simulink model "lab_1"  (R2024b)
settings: Solver=FixedStepAuto  StartTime=0.0  StopTime=inf  FixedStep=0.001  RelTol=1e-3  EnableMultiTasking=on
libraries: stm32f4xxblockslib x16, simulink x15, stm32g4xxblockslib x6
settings Model: STM32="{\"AnalogInput\":[{\"ID\":\"lab_1:1\"},{\"ID\":\"lab_1:151\"},{\"ID\":\"lab_1:191\"}],\"DigitalPortRead\":[{\"ID\":\"lab_1:126\"},{\"ID\":\"lab_1:163\"},{\"ID\":\"lab_1:197\"},{\"ID\":\"lab_1:248\"},{\"ID\":\"lab_1:260\"},{\"ID\":\"lab_1:272\"},{\"ID\":\"lab_1:237\"},{\"ID\":\"lab_1:238\"},{\"ID\":\"lab_1:303\"},{\"ID\":\"lab_1:314\"},{\"ID\":\"lab_1:325\"},{\"ID\":\"lab_1:293\"},{\"ID\":\"lab_1:294\"}],\"EncoderBlockForG4\":[{\"ID\":\"lab_1:234\"},{\"ID\":\"lab_1:235\"},{\"ID\":\"lab_1:236\"},{\"ID\":\"lab_1:290\"},{\"ID\":\"lab_1:291\"},{\"ID\":\"lab_1:292\"}]}"  Creator=A1nz_01  LastModifiedBy=user
settings OptimizationCC: EnhancedBackFolding=on  PassReuseOutputArgsAs=Individual arguments  ZeroExternalMemoryAtStartup=off  ZeroInternalMemoryAtStartup=off  MaxStackSize=512  OptimizeBlockOrder=speed  DifferentSizesBufferReuse=on  OptimizationCustomize=off  EfficientTunableParamExpr=on
settings DebuggingCC: ParameterTunabilityLossMsg=error
settings HardwareCC: ProdBitPerPointer=32  ProdBitPerSizeT=32  ProdBitPerPtrDiffT=32  ProdLargestAtomicInteger=Long  ProdLargestAtomicFloat=Double  ProdWordSize=32  ProdLongLongMode=on  ProdHWDeviceType=ARM Compatible->ARM Cortex-M
settings SFSimCC: MATLABDynamicMemAlloc=off
settings RTWCC: Description=Embedded Coder  SystemTargetFile=ert.tlc  HardwareBoard=STM32G4xx Based  TemplateMakefile=ert_default_tmf  Toolchain=GNU Tools for ARM Embedded Processors
settings CodeAppCC: ForceParamTrailComments=on  IgnoreCustomStorageClasses=off  OperatorAnnotations=on  SimulinkDataObjDesc=on  SFDataObjDesc=on  InsertBlockDesc=on
settings ERTTargetCC: TargetLangStandard=C99 (ISO)  CodeReplacementLibrary=ARM Cortex-M  ExtModeTransport=3  ExtModeStaticAlloc=on  ExtModeStaticAllocSize=2048  ExtModeMexFile=ext_xcp  ExtModeIntrfLevel=Level2 - Open  InlinedParameterPlacement=Hierarchical  DynamicArrayContainerType=coder::array

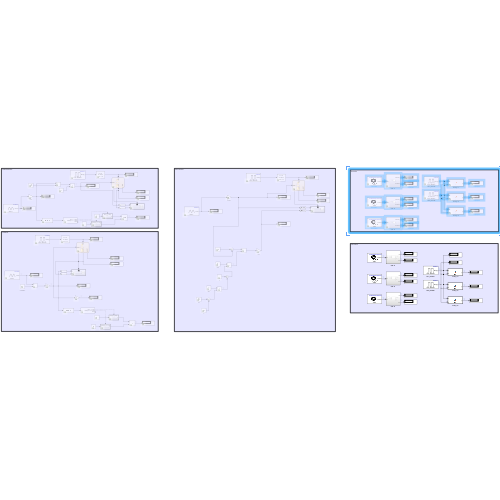
[thumbnail: Simulink's stored preview of the top-level diagram]
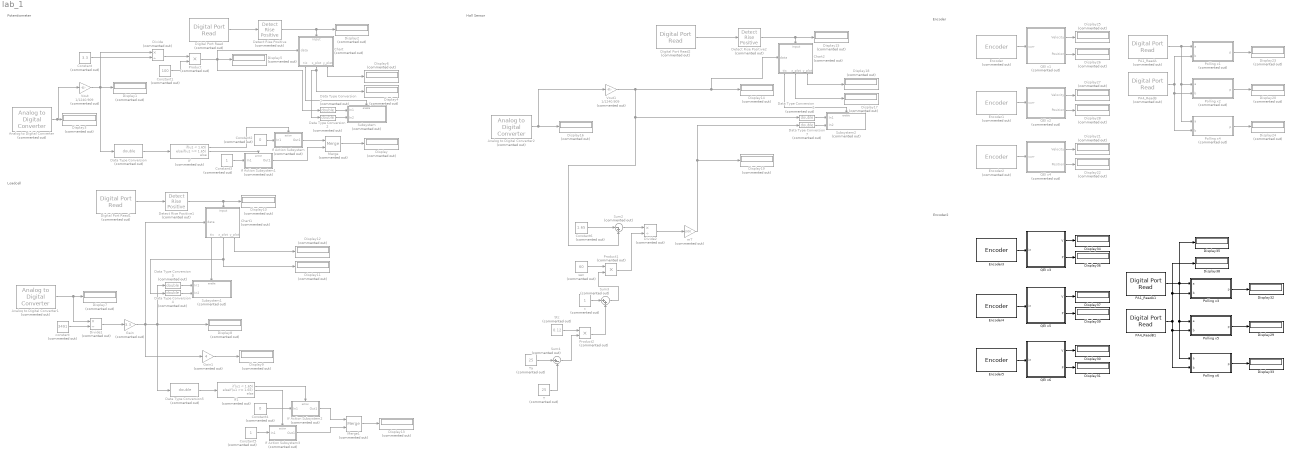
== system lab_1 ==
  note: Encoder2
  note: Encoder
  note: Hall Sensor
  note: Loadcell
  note: Potentiometer
  Analog to Digital Converter : stm32f4xxblockslib/Analog to Digital Converter  Commented=on  ADCModule=ADC1  ConversionGroup=Regular  TriggerMode=Trigger and read  NumberOfConversions=1  EnableBufferConv=off  BufferLength=1  OutputStatus=off  SampleTime=-1  EnableSimPort=off  hoistedMaskSrc=ECSoC/ECSimCodegen/Analog to Digital Converter
  Analog to Digital Converter1 : stm32f4xxblockslib/Analog to Digital Converter  Commented=on  ADCModule=ADC1  ConversionGroup=Regular  TriggerMode=Trigger and read  NumberOfConversions=1  EnableBufferConv=off  BufferLength=1  OutputStatus=off  SampleTime=-1  EnableSimPort=off  hoistedMaskSrc=ECSoC/ECSimCodegen/Analog to Digital Converter
  Analog to Digital Converter2 : stm32f4xxblockslib/Analog to Digital Converter  Commented=on  ADCModule=ADC1  ConversionGroup=Regular  TriggerMode=Trigger and read  NumberOfConversions=1  EnableBufferConv=off  BufferLength=1  OutputStatus=off  SampleTime=-1  EnableSimPort=off  hoistedMaskSrc=ECSoC/ECSimCodegen/Analog to Digital Converter
  Chart : Stateflow chart  Commented=on  TreatAsAtomicUnit=on
      settings: PortSchema="{\"entries\":[{\"content\":{\"sides\":[{\"content\":{\"connectorIds\":[\"In1\"]},\"type\":\"ConnectorPlacement.EquallySpacedRectSide\",\"uuid\":\"15421bba-938f-45a9-ad39-0fb1dc31f746\"},{\"content\":{\"side\":\"RIGHT\"},\"type\":\"ConnectorPlacement.EquallySpacedRectSide\",\"uuid\":\"6df644a9-cb47-4d86-919b-b55e97b0d3b9\"},{\"content\":{\"connectorIds\":[\"In2\"],\"side\":\"TOP\"},\"type\":\"ConnectorPlacement.EquallySpacedRectSide\",\"uuid\":\"9fcc37fd-4916-48d6-817c-74b5556d6fa8\"},{\"content\":{\"connectorIds\":[\"Out1\",\"Out2\",\"Out3\"],\"side\":\"BOTTOM\"},\"type\":\"ConnectorPlacement.EquallySpacedRectSide\",\"uuid\":\"cb540dc6-d65e-4d03-87d2-789e1aed4831\"}]},\"type\":\"ConnectorPlacement.EquallySpacedConnector\",\"uuid\":\"c07b23df-6d95-4e9d-8fab-891c31dfc579\"}],\"packageUris\":[\"http://schema.mathworks.com/mf0/Connector/R2020b\"],\"version\":\"1.0\"}"
  Chart1 : Stateflow chart  Commented=on  TreatAsAtomicUnit=on
      settings: PortSchema="{\"entries\":[{\"content\":{\"sides\":[{\"content\":{\"connectorIds\":[\"In1\"]},\"type\":\"ConnectorPlacement.EquallySpacedRectSide\",\"uuid\":\"15421bba-938f-45a9-ad39-0fb1dc31f746\"},{\"content\":{\"side\":\"RIGHT\"},\"type\":\"ConnectorPlacement.EquallySpacedRectSide\",\"uuid\":\"6df644a9-cb47-4d86-919b-b55e97b0d3b9\"},{\"content\":{\"connectorIds\":[\"In2\"],\"side\":\"TOP\"},\"type\":\"ConnectorPlacement.EquallySpacedRectSide\",\"uuid\":\"9fcc37fd-4916-48d6-817c-74b5556d6fa8\"},{\"content\":{\"connectorIds\":[\"Out1\",\"Out2\",\"Out3\"],\"side\":\"BOTTOM\"},\"type\":\"ConnectorPlacement.EquallySpacedRectSide\",\"uuid\":\"cb540dc6-d65e-4d03-87d2-789e1aed4831\"}]},\"type\":\"ConnectorPlacement.EquallySpacedConnector\",\"uuid\":\"c07b23df-6d95-4e9d-8fab-891c31dfc579\"}],\"packageUris\":[\"http://schema.mathworks.com/mf0/Connector/R2020b\"],\"version\":\"1.0\"}"
  Chart2 : Stateflow chart  Commented=on  TreatAsAtomicUnit=on
      settings: PortSchema="{\"entries\":[{\"content\":{\"sides\":[{\"content\":{\"connectorIds\":[\"In1\"]},\"type\":\"ConnectorPlacement.EquallySpacedRectSide\",\"uuid\":\"15421bba-938f-45a9-ad39-0fb1dc31f746\"},{\"content\":{\"side\":\"RIGHT\"},\"type\":\"ConnectorPlacement.EquallySpacedRectSide\",\"uuid\":\"6df644a9-cb47-4d86-919b-b55e97b0d3b9\"},{\"content\":{\"connectorIds\":[\"In2\"],\"side\":\"TOP\"},\"type\":\"ConnectorPlacement.EquallySpacedRectSide\",\"uuid\":\"9fcc37fd-4916-48d6-817c-74b5556d6fa8\"},{\"content\":{\"connectorIds\":[\"Out1\",\"Out2\",\"Out3\"],\"side\":\"BOTTOM\"},\"type\":\"ConnectorPlacement.EquallySpacedRectSide\",\"uuid\":\"cb540dc6-d65e-4d03-87d2-789e1aed4831\"}]},\"type\":\"ConnectorPlacement.EquallySpacedConnector\",\"uuid\":\"c07b23df-6d95-4e9d-8fab-891c31dfc579\"}],\"packageUris\":[\"http://schema.mathworks.com/mf0/Connector/R2020b\"],\"version\":\"1.0\"}"
  Constant : Constant  Commented=on  Value=3.3
  Constant1 : Constant  Commented=on  Value=100
  Constant2 : Constant  Commented=on  Value=0
  Constant3 : Constant  Commented=on
  Constant4 : Constant  Commented=on  Value=0
  Constant5 : Constant  Commented=on
  Constant6 : Constant  Commented=on  Value=1.65
  Data Type Conversion{,1..7} (8 alike) : DataTypeConversion  Commented=on  OutDataTypeStr=double  SaturateOnIntegerOverflow=off  RndMeth=Floor
  Detect Rise Positive : simulink/Logic and Bit Operations/Detect Rise Positive  Commented=on  vinit=0  OutDataTypeStr=boolean
  Detect Rise Positive1 : simulink/Logic and Bit Operations/Detect Rise Positive  Commented=on  vinit=0  OutDataTypeStr=boolean
  Detect Rise Positive2 : simulink/Logic and Bit Operations/Detect Rise Positive  Commented=on  vinit=0  OutDataTypeStr=boolean
  Digital Port Read : stm32f4xxblockslib/Digital Port Read  Commented=on  PortName=GPIOC  PinNumber=[13]  ReadOperation=on  IOAsArray=on  SampleTime=-1  EnableSimPort=off  hoistedMaskSrc=ECSoC/ECSimCodegen/Digital Port Read
      settings: LibrarySourceBlock=stm32g4xxblockslib/Digital Port Read
  Digital Port Read1 : stm32f4xxblockslib/Digital Port Read  Commented=on  PortName=GPIOC  PinNumber=[13]  ReadOperation=on  IOAsArray=on  SampleTime=-1  EnableSimPort=off  hoistedMaskSrc=ECSoC/ECSimCodegen/Digital Port Read
      settings: LibrarySourceBlock=stm32g4xxblockslib/Digital Port Read
  Digital Port Read2 : stm32f4xxblockslib/Digital Port Read  Commented=on  PortName=GPIOC  PinNumber=[13]  ReadOperation=on  IOAsArray=on  SampleTime=-1  EnableSimPort=off  hoistedMaskSrc=ECSoC/ECSimCodegen/Digital Port Read
      settings: LibrarySourceBlock=stm32g4xxblockslib/Digital Port Read
  Display{,1..28} (29 alike) : Display  Commented=on
  Display{29..39} (11 alike) : Display
  Divide : Product  Commented=on  Inputs=*/
  Divide1 : Product  Commented=on  Inputs=*/
  Divide2 : Product  Commented=on  Inputs=*/
  Encoder : stm32g4xxblockslib/Encoder  Commented=on  TimerModule=TIM1  EnableResetInput=off  OutputCountAfterFirstIndex=off  OutputValidIndex=off  OutputDirection=off  OutputStatus=off  SampleTime=-1
  Encoder1 : stm32g4xxblockslib/Encoder  Commented=on  TimerModule=TIM4  EnableResetInput=off  OutputCountAfterFirstIndex=off  OutputValidIndex=off  OutputDirection=off  OutputStatus=off  SampleTime=-1
  Encoder2 : stm32g4xxblockslib/Encoder  Commented=on  TimerModule=TIM3  EnableResetInput=off  OutputCountAfterFirstIndex=off  OutputValidIndex=off  OutputDirection=off  OutputStatus=off  SampleTime=-1
  Encoder3 : stm32g4xxblockslib/Encoder  TimerModule=TIM1  EnableResetInput=off  OutputCountAfterFirstIndex=off  OutputValidIndex=off  OutputDirection=off  OutputStatus=off  SampleTime=-1
  Encoder4 : stm32g4xxblockslib/Encoder  TimerModule=TIM4  EnableResetInput=off  OutputCountAfterFirstIndex=off  OutputValidIndex=off  OutputDirection=off  OutputStatus=off  SampleTime=-1
  Encoder5 : stm32g4xxblockslib/Encoder  TimerModule=TIM3  EnableResetInput=off  OutputCountAfterFirstIndex=off  OutputValidIndex=off  OutputDirection=off  OutputStatus=off  SampleTime=-1
  Gain : Gain  Commented=on  Gain=3.3
  Gain1 : Gain  Commented=on  Gain=4
  If : If  Commented=on  IfExpression=u1 < 1.65  ElseIfExpressions=u1 >= 1.65
  If Action Subsystem : Subsystem  Commented=on  TreatAsAtomicUnit=on
  If Action Subsystem1 : Subsystem  Commented=on  TreatAsAtomicUnit=on
  If Action Subsystem2 : Subsystem  Commented=on  TreatAsAtomicUnit=on
  If Action Subsystem3 : Subsystem  Commented=on  TreatAsAtomicUnit=on
  If1 : If  Commented=on  IfExpression=u1 < 1.65  ElseIfExpressions=u1 >= 1.65
  Merge : Merge  Commented=on
  Merge1 : Merge  Commented=on
  PA1_ReadA : stm32f4xxblockslib/Digital Port Read  Commented=on  PortName=GPIOA  PinNumber=[1]  ReadOperation=on  IOAsArray=on  SampleTime=-1  EnableSimPort=off  hoistedMaskSrc=ECSoC/ECSimCodegen/Digital Port Read
      settings: LibrarySourceBlock=stm32g4xxblockslib/Digital Port Read
  PA1_ReadA1 : stm32f4xxblockslib/Digital Port Read  PortName=GPIOA  PinNumber=[1]  ReadOperation=on  IOAsArray=on  SampleTime=-1  EnableSimPort=off  hoistedMaskSrc=ECSoC/ECSimCodegen/Digital Port Read
      settings: LibrarySourceBlock=stm32g4xxblockslib/Digital Port Read
  PA4_ReadB : stm32f4xxblockslib/Digital Port Read  Commented=on  PortName=GPIOA  PinNumber=[4]  ReadOperation=on  IOAsArray=on  SampleTime=-1  EnableSimPort=off  hoistedMaskSrc=ECSoC/ECSimCodegen/Digital Port Read
      settings: LibrarySourceBlock=stm32g4xxblockslib/Digital Port Read
  PA4_ReadB1 : stm32f4xxblockslib/Digital Port Read  PortName=GPIOA  PinNumber=[4]  ReadOperation=on  IOAsArray=on  SampleTime=-1  EnableSimPort=off  hoistedMaskSrc=ECSoC/ECSimCodegen/Digital Port Read
      settings: LibrarySourceBlock=stm32g4xxblockslib/Digital Port Read
  Polling x1 : MATLAB Function  Commented=on  TreatAsAtomicUnit=on
  Polling x2 : MATLAB Function  Commented=on  TreatAsAtomicUnit=on
  Polling x3 : MATLAB Function  TreatAsAtomicUnit=on
  Polling x4 : MATLAB Function  Commented=on  TreatAsAtomicUnit=on
  Polling x5 : MATLAB Function  TreatAsAtomicUnit=on
  Polling x6 : MATLAB Function  TreatAsAtomicUnit=on
  Product : Product  Commented=on
  Product1 : Product  Commented=on
  Product2 : Product  Commented=on
  QEI x1 : Subsystem  Commented=on
  QEI x2 : Subsystem  Commented=on
  QEI x3 : Subsystem
  QEI x4 : Subsystem  Commented=on
  QEI x5 : Subsystem
  QEI x6 : Subsystem
  Stc : Constant  Commented=on  Value=0.12
  Subsystem : Subsystem  Commented=on
  Subsystem1 : Subsystem  Commented=on
  Subsystem2 : Subsystem  Commented=on
  Sum2 : Sum  Commented=on  Inputs=|-+
  Sum3 : Sum  Commented=on  Inputs=|++
  Sum4 : Sum  Commented=on  Inputs=|+-
  T : Constant  Commented=on  Value=25
  Ta : Constant  Commented=on  Value=25
  Vout : Gain  Commented=on  Gain=1/1240.909
  Vout1 : Gain  Commented=on  Gain=1/1240.909
  c : Constant  Commented=on
  constant : Constant  Commented=on  Value=3491
  mT : Gain  Commented=on  Gain=1000
  sen : Constant  Commented=on  Value=60
  wires:
  Analog to Digital Converter/1 -> Vout/1, Display3/1
  Constant/1 -> Divide/2
  Divide/1 -> Product/1
  Constant1/1 -> Product/2
  Product/1 -> Data Type Conversion1/1, Chart/1(data), Display5/1
  Vout/1 -> Divide/1, Display1/1, Data Type Conversion/1
  Constant2/1 -> If Action Subsystem/1(In1)
  Data Type Conversion/1 -> If/1
  If/1 -> If Action Subsystem/Action
  If/2 -> If Action Subsystem1/Action
  Constant3/1 -> If Action Subsystem1/1(In1)
  If Action Subsystem/1(Out1) -> Merge/1
  If Action Subsystem1/1(Out1) -> Merge/2
  Merge/1 -> Display/1
  Digital Port Read/1 -> Detect Rise Positive/1
  Detect Rise Positive/1 -> Display2/1, Chart/2(input)
  Data Type Conversion1/1 -> Subsystem/1(In1)
  Data Type Conversion2/1 -> Subsystem/2(In2)
  Chart/1(tic) -> Subsystem/Enable
  Chart/2(x_plot) -> Data Type Conversion2/1, Display4/1
  Chart/3(y_plot) -> Display6/1
  Divide1/1 -> Gain/1
  constant/1 -> Divide1/2
  Analog to Digital Converter1/1 -> Divide1/1, Display7/1
  Gain1/1 -> Display9/1
  Detect Rise Positive1/1 -> Display10/1, Chart1/2(input)
  Digital Port Read1/1 -> Detect Rise Positive1/1
  Chart1/3(y_plot) -> Display12/1
  Gain/1 -> Chart1/1(data), Gain1/1, Data Type Conversion5/1, Display8/1, Data Type Conversion3/1
  Data Type Conversion4/1 -> Subsystem1/2(In2)
  Chart1/1(tic) -> Subsystem1/Enable
  Chart1/2(x_plot) -> Data Type Conversion4/1, Display11/1
  Data Type Conversion3/1 -> Subsystem1/1(In1)
  If1/1 -> If Action Subsystem2/Action
  Constant4/1 -> If Action Subsystem2/1(In1)
  If Action Subsystem2/1(Out1) -> Merge1/1
  Constant5/1 -> If Action Subsystem3/1(In1)
  If Action Subsystem3/1(Out1) -> Merge1/2
  If1/2 -> If Action Subsystem3/Action
  Data Type Conversion5/1 -> If1/1
  Merge1/1 -> Display13/1
  Sum3/1 -> Product1/2
  Sum4/1 -> Product2/2
  Stc/1 -> Product2/1
  Ta/1 -> Sum4/1
  Data Type Conversion7/1 -> Subsystem2/2(In2)
  mT/1 -> Display19/1, Data Type Conversion7/1
  Divide2/1 -> mT/1
  Vout1/1 -> Chart2/1(data), Display14/1, Data Type Conversion6/1, Sum2/2
  Chart2/2(x_plot) -> Display17/1
  c/1 -> Sum3/1
  sen/1 -> Product1/1
  Analog to Digital Converter2/1 -> Vout1/1, Display16/1
  Product2/1 -> Sum3/2
  Detect Rise Positive2/1 -> Display15/1, Chart2/2(input)
  Product1/1 -> Divide2/2
  Data Type Conversion6/1 -> Subsystem2/1(In1)
  T/1 -> Sum4/2
  Digital Port Read2/1 -> Detect Rise Positive2/1
  Constant6/1 -> Sum2/1
  Chart2/3(y_plot) -> Display18/1
  Sum2/1 -> Divide2/1
  Chart2/1(tic) -> Subsystem2/Enable
  QEI x4/2(Position) -> Display22/1
  Polling x2/1(p) -> Display20/1
  QEI x4/1(Velocity) -> Display21/1
  QEI x1/1(Velocity) -> Display25/1
  PA4_ReadB/1 -> Polling x2/2(b), Polling x4/2(b), Polling x1/2(b)
  Encoder2/1 -> QEI x4/1(curr)
  Polling x4/1(p) -> Display24/1
  QEI x1/2(Position) -> Display26/1
  PA1_ReadA/1 -> Polling x4/1(a), Polling x2/1(a), Polling x1/1(a)
  Polling x1/1(p) -> Display23/1
  QEI x2/2(Position) -> Display28/1
  Encoder1/1 -> QEI x2/1(curr)
  QEI x2/1(Velocity) -> Display27/1
  Encoder/1 -> QEI x1/1(curr)
  QEI x5/1(V) -> Display37/1
  Encoder4/1 -> QEI x5/1(in)
  QEI x3/1(V) -> Display34/1
  QEI x6/1(V) -> Display30/1
  QEI x3/2(P) -> Display36/1
  Polling x5/1(p) -> Display29/1
  Encoder3/1 -> QEI x3/1(in)
  Polling x3/1(p) -> Display32/1
  QEI x6/2(P) -> Display31/1
  QEI x5/2(P) -> Display39/1
  Encoder5/1 -> QEI x6/1(in)
  Polling x6/1(p) -> Display33/1
  PA1_ReadA1/1 -> Display35/1, Polling x6/1(a), Polling x5/1(a), Polling x3/1(a)
  PA4_ReadB1/1 -> Polling x5/2(b), Polling x6/2(b), Display38/1, Polling x3/2(b)

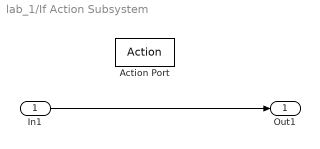
== system lab_1/If Action Subsystem ==
  In1 : Inport
  Action Port : ActionPort  ActionPortLabel=if(u1 < 1.65)
  Out1 : Outport
  wires:
  In1/1 -> Out1/1

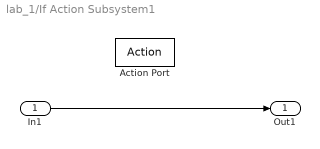
== system lab_1/If Action Subsystem1 ==
  In1 : Inport
  Action Port : ActionPort  ActionPortLabel=elseif(u1 >= 1.65)
  Out1 : Outport
  wires:
  In1/1 -> Out1/1

== system lab_1/If Action Subsystem2 ==
  In1 : Inport
  Action Port : ActionPort  ActionPortLabel=if(u1 < 1.65)
  Out1 : Outport
  wires:
  In1/1 -> Out1/1

== system lab_1/If Action Subsystem3 ==
  In1 : Inport
  Action Port : ActionPort  ActionPortLabel=elseif(u1 >= 1.65)
  Out1 : Outport
  wires:
  In1/1 -> Out1/1

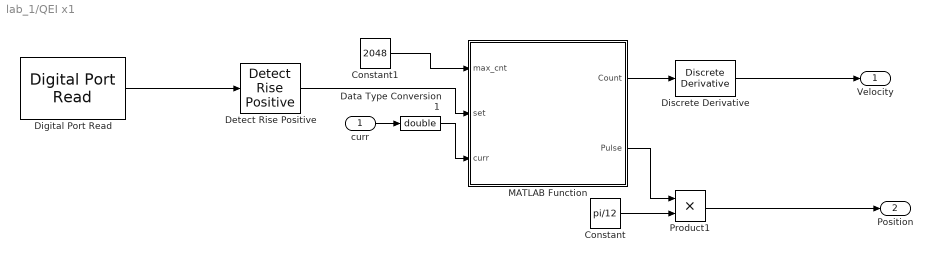
== system lab_1/QEI x1 ==
  curr : Inport
  Constant : Constant  Value=pi/12
  Constant1 : Constant  Value=2048
  Data Type Conversion1 : DataTypeConversion  OutDataTypeStr=double  SaturateOnIntegerOverflow=off  RndMeth=Floor
  Detect Rise Positive : simulink/Logic and Bit Operations/Detect Rise Positive  vinit=0  OutDataTypeStr=boolean
  Digital Port Read : stm32f4xxblockslib/Digital Port Read  PortName=GPIOC  PinNumber=[13]  ReadOperation=on  IOAsArray=on  SampleTime=-1  EnableSimPort=off  hoistedMaskSrc=ECSoC/ECSimCodegen/Digital Port Read
      settings: LibrarySourceBlock=stm32g4xxblockslib/Digital Port Read
  Discrete Derivative : simulink/Discrete/Discrete Derivative  gainval=1.0  ICPrevScaledInput=0.0  OutMin=[]  OutMax=[]  OutDataType=fixdt(1, 16)  OutScaling=2^-10  DoSatur=off
  MATLAB Function : MATLAB Function  TreatAsAtomicUnit=on
  Product1 : Product
  Velocity : Outport
  Position : Outport  Port=2
  wires:
  Digital Port Read/1 -> Detect Rise Positive/1
  Detect Rise Positive/1 -> MATLAB Function/2(set)
  Data Type Conversion1/1 -> MATLAB Function/3(curr)
  curr/1 -> Data Type Conversion1/1
  MATLAB Function/1(Count) -> Discrete Derivative/1
  Discrete Derivative/1 -> Velocity/1
  MATLAB Function/2(Pulse) -> Product1/1
  Constant/1 -> Product1/2
  Product1/1 -> Position/1
  Constant1/1 -> MATLAB Function/1(max_cnt)

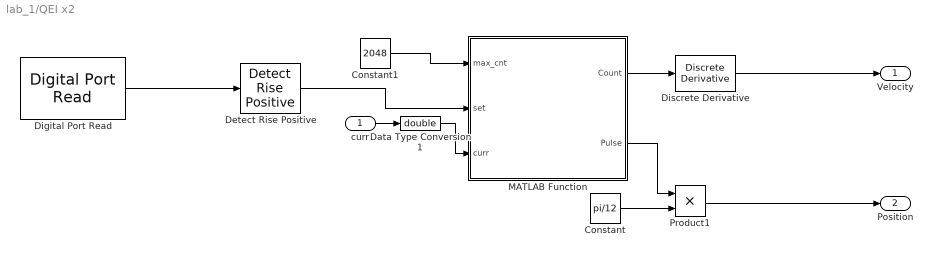
== system lab_1/QEI x2 ==
  curr : Inport
  Constant : Constant  Value=pi/12
  Constant1 : Constant  Value=2048
  Data Type Conversion1 : DataTypeConversion  OutDataTypeStr=double  SaturateOnIntegerOverflow=off  RndMeth=Floor
  Detect Rise Positive : simulink/Logic and Bit Operations/Detect Rise Positive  vinit=0  OutDataTypeStr=boolean
  Digital Port Read : stm32f4xxblockslib/Digital Port Read  PortName=GPIOC  PinNumber=[13]  ReadOperation=on  IOAsArray=on  SampleTime=-1  EnableSimPort=off  hoistedMaskSrc=ECSoC/ECSimCodegen/Digital Port Read
  Discrete Derivative : simulink/Discrete/Discrete Derivative  gainval=1.0  ICPrevScaledInput=0.0  OutMin=[]  OutMax=[]  OutDataType=fixdt(1, 16)  OutScaling=2^-10  DoSatur=off
  MATLAB Function : MATLAB Function  TreatAsAtomicUnit=on
  Product1 : Product
  Velocity : Outport
  Position : Outport  Port=2
  wires:
  Digital Port Read/1 -> Detect Rise Positive/1
  Detect Rise Positive/1 -> MATLAB Function/2(set)
  Data Type Conversion1/1 -> MATLAB Function/3(curr)
  curr/1 -> Data Type Conversion1/1
  MATLAB Function/1(Count) -> Discrete Derivative/1
  Discrete Derivative/1 -> Velocity/1
  MATLAB Function/2(Pulse) -> Product1/1
  Constant/1 -> Product1/2
  Product1/1 -> Position/1
  Constant1/1 -> MATLAB Function/1(max_cnt)

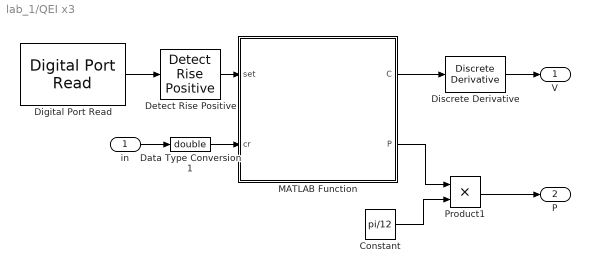
== system lab_1/QEI x3 ==
  in : Inport
  Constant : Constant  Value=pi/12
  Data Type Conversion1 : DataTypeConversion  OutDataTypeStr=double  SaturateOnIntegerOverflow=off  RndMeth=Floor
  Detect Rise Positive : simulink/Logic and Bit Operations/Detect Rise Positive  vinit=0  OutDataTypeStr=boolean
  Digital Port Read : stm32f4xxblockslib/Digital Port Read  PortName=GPIOC  PinNumber=[13]  ReadOperation=on  IOAsArray=on  SampleTime=-1  EnableSimPort=off  hoistedMaskSrc=ECSoC/ECSimCodegen/Digital Port Read
      settings: LibrarySourceBlock=stm32g4xxblockslib/Digital Port Read
  Discrete Derivative : simulink/Discrete/Discrete Derivative  gainval=1.0  ICPrevScaledInput=0.0  OutMin=[]  OutMax=[]  OutDataType=fixdt(1, 16)  OutScaling=2^-10  DoSatur=off
  MATLAB Function : MATLAB Function  TreatAsAtomicUnit=on
  Product1 : Product
  V : Outport
  P : Outport  Port=2
  wires:
  Digital Port Read/1 -> Detect Rise Positive/1
  Detect Rise Positive/1 -> MATLAB Function/1(set)
  Data Type Conversion1/1 -> MATLAB Function/2(cr)
  in/1 -> Data Type Conversion1/1
  MATLAB Function/1(C) -> Discrete Derivative/1
  Discrete Derivative/1 -> V/1
  MATLAB Function/2(P) -> Product1/1
  Constant/1 -> Product1/2
  Product1/1 -> P/1

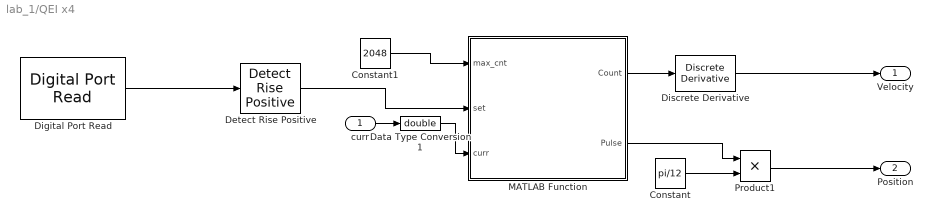
== system lab_1/QEI x4 ==
  curr : Inport
  Constant : Constant  Value=pi/12
  Constant1 : Constant  Value=2048
  Data Type Conversion1 : DataTypeConversion  OutDataTypeStr=double  SaturateOnIntegerOverflow=off  RndMeth=Floor
  Detect Rise Positive : simulink/Logic and Bit Operations/Detect Rise Positive  vinit=0  OutDataTypeStr=boolean
  Digital Port Read : stm32f4xxblockslib/Digital Port Read  PortName=GPIOC  PinNumber=[13]  ReadOperation=on  IOAsArray=on  SampleTime=-1  EnableSimPort=off  hoistedMaskSrc=ECSoC/ECSimCodegen/Digital Port Read
  Discrete Derivative : simulink/Discrete/Discrete Derivative  gainval=1.0  ICPrevScaledInput=0.0  OutMin=[]  OutMax=[]  OutDataType=fixdt(1, 16)  OutScaling=2^-10  DoSatur=off
  MATLAB Function : MATLAB Function  TreatAsAtomicUnit=on
  Product1 : Product
  Velocity : Outport
  Position : Outport  Port=2
  wires:
  Digital Port Read/1 -> Detect Rise Positive/1
  Detect Rise Positive/1 -> MATLAB Function/2(set)
  Data Type Conversion1/1 -> MATLAB Function/3(curr)
  curr/1 -> Data Type Conversion1/1
  MATLAB Function/1(Count) -> Discrete Derivative/1
  Discrete Derivative/1 -> Velocity/1
  MATLAB Function/2(Pulse) -> Product1/1
  Constant/1 -> Product1/2
  Product1/1 -> Position/1
  Constant1/1 -> MATLAB Function/1(max_cnt)

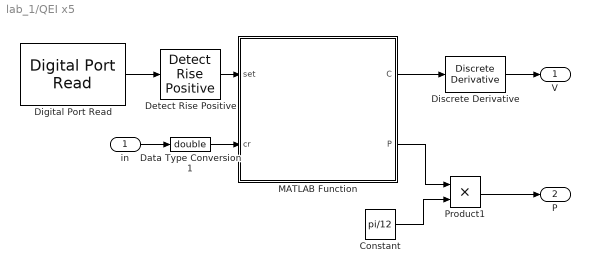
== system lab_1/QEI x5 ==
  in : Inport
  Constant : Constant  Value=pi/12
  Data Type Conversion1 : DataTypeConversion  OutDataTypeStr=double  SaturateOnIntegerOverflow=off  RndMeth=Floor
  Detect Rise Positive : simulink/Logic and Bit Operations/Detect Rise Positive  vinit=0  OutDataTypeStr=boolean
  Digital Port Read : stm32f4xxblockslib/Digital Port Read  PortName=GPIOC  PinNumber=[13]  ReadOperation=on  IOAsArray=on  SampleTime=-1  EnableSimPort=off  hoistedMaskSrc=ECSoC/ECSimCodegen/Digital Port Read
  Discrete Derivative : simulink/Discrete/Discrete Derivative  gainval=1.0  ICPrevScaledInput=0.0  OutMin=[]  OutMax=[]  OutDataType=fixdt(1, 16)  OutScaling=2^-10  DoSatur=off
  MATLAB Function : MATLAB Function  TreatAsAtomicUnit=on
  Product1 : Product
  V : Outport
  P : Outport  Port=2
  wires:
  Digital Port Read/1 -> Detect Rise Positive/1
  Detect Rise Positive/1 -> MATLAB Function/1(set)
  Data Type Conversion1/1 -> MATLAB Function/2(cr)
  in/1 -> Data Type Conversion1/1
  MATLAB Function/1(C) -> Discrete Derivative/1
  Discrete Derivative/1 -> V/1
  MATLAB Function/2(P) -> Product1/1
  Constant/1 -> Product1/2
  Product1/1 -> P/1

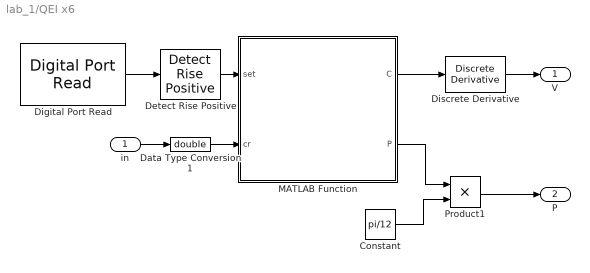
== system lab_1/QEI x6 ==
  in : Inport
  Constant : Constant  Value=pi/12
  Data Type Conversion1 : DataTypeConversion  OutDataTypeStr=double  SaturateOnIntegerOverflow=off  RndMeth=Floor
  Detect Rise Positive : simulink/Logic and Bit Operations/Detect Rise Positive  vinit=0  OutDataTypeStr=boolean
  Digital Port Read : stm32f4xxblockslib/Digital Port Read  PortName=GPIOC  PinNumber=[13]  ReadOperation=on  IOAsArray=on  SampleTime=-1  EnableSimPort=off  hoistedMaskSrc=ECSoC/ECSimCodegen/Digital Port Read
  Discrete Derivative : simulink/Discrete/Discrete Derivative  gainval=1.0  ICPrevScaledInput=0.0  OutMin=[]  OutMax=[]  OutDataType=fixdt(1, 16)  OutScaling=2^-10  DoSatur=off
  MATLAB Function : MATLAB Function  TreatAsAtomicUnit=on
  Product1 : Product
  V : Outport
  P : Outport  Port=2
  wires:
  Digital Port Read/1 -> Detect Rise Positive/1
  Detect Rise Positive/1 -> MATLAB Function/1(set)
  Data Type Conversion1/1 -> MATLAB Function/2(cr)
  in/1 -> Data Type Conversion1/1
  MATLAB Function/1(C) -> Discrete Derivative/1
  Discrete Derivative/1 -> V/1
  MATLAB Function/2(P) -> Product1/1
  Constant/1 -> Product1/2
  Product1/1 -> P/1

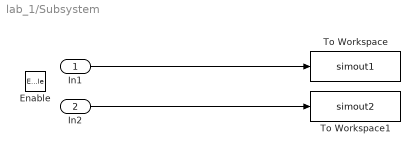
== system lab_1/Subsystem ==
  In1 : Inport
  In2 : Inport  Port=2
  Enable : EnablePort
  To Workspace : ToWorkspace  VariableName=simout1  SampleTime=-1
      settings: Save2DSignal=2-D array (concatenate along first dimension)
  To Workspace1 : ToWorkspace  VariableName=simout2  SampleTime=-1
      settings: Save2DSignal=2-D array (concatenate along first dimension)
  wires:
  In1/1 -> To Workspace/1
  In2/1 -> To Workspace1/1

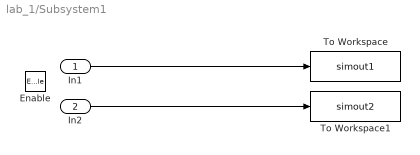
== system lab_1/Subsystem1 ==
  In1 : Inport
  In2 : Inport  Port=2
  Enable : EnablePort
  To Workspace : ToWorkspace  VariableName=simout1  SampleTime=-1
      settings: Save2DSignal=2-D array (concatenate along first dimension)
  To Workspace1 : ToWorkspace  VariableName=simout2  SampleTime=-1
      settings: Save2DSignal=2-D array (concatenate along first dimension)
  wires:
  In1/1 -> To Workspace/1
  In2/1 -> To Workspace1/1

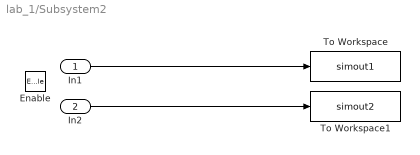
== system lab_1/Subsystem2 ==
  In1 : Inport
  In2 : Inport  Port=2
  Enable : EnablePort
  To Workspace : ToWorkspace  VariableName=simout1  SampleTime=-1
      settings: Save2DSignal=2-D array (concatenate along first dimension)
  To Workspace1 : ToWorkspace  VariableName=simout2  SampleTime=-1
      settings: Save2DSignal=2-D array (concatenate along first dimension)
  wires:
  In1/1 -> To Workspace/1
  In2/1 -> To Workspace1/1

== matlab function lab_1/QEI x2/MATLAB Function ==
  data: max_cnt input; Count output; Pulse output; set input; curr input
function [Count,Pulse] = fcn(max_cnt,set,curr)
    persistent prev;
    persistent homing;
    persistent pos;

    if isempty(prev)
        prev = curr;
        homing = 0;
        pos = 0;
    end

    delta = curr - prev;

    if delta <= -1*(max_cnt/2)
        delta = delta + max_cnt + 1;
    elseif delta >= max_cnt/2
        delta = delta -max_cnt - 1;
    end

    if set
        homing = pos;
    end

    pos = pos + delta;
    Count = pos - homing;
    prev = curr;

    Pulse = Count;

end

== matlab function lab_1/QEI x4/MATLAB Function ==
  data: max_cnt input; Count output; Pulse output; set input; curr input
function [Count,Pulse] = fcn(max_cnt,set,curr)
    persistent prev;
    persistent homing;
    persistent pos;

    if isempty(prev)
        prev = curr;
        homing = 0;
        pos = 0;
    end

    delta = curr - prev;

    if delta <= -1*(max_cnt/2)
        delta = delta + max_cnt + 1;
    elseif delta >= max_cnt/2
        delta = delta -max_cnt - 1;
    end

    if set
        homing = pos;
    end

    pos = pos + delta;
    Count = pos - homing;
    prev = curr;

    Pulse = Count;

end

== matlab function lab_1/Polling x3 ==
  data: a input; p output; b input
function p = fcn(a,b)
    persistent pos;
    persistent trig;
    if isempty(trig)
        trig = 1;
        pos = 0;
    end
    if a-b == -1 && trig
        pos = pos + 1;
        trig = 0;
    elseif a-b == 1 && trig
        pos = pos -1;
        trig = 0;
    end

    if a == 1 && b == 1
        trig = 1;
    end
    p = pos;
end

== matlab function lab_1/Polling x5 ==
  data: a input; p output; b input
function p = fcn(a,b)
    persistent pos;
    persistent trig;
    if isempty(trig)
        trig = 1;
        pos = 0;
    end
    if a-b == -1 && trig
        pos = pos + 1;
        trig = 2;
    elseif a-b == 1 && trig
        pos = pos -1;
        trig = 2;
    end

    if a == 0 && b == 0 
        trig = 0;
    end

    if a-b == 1 && trig == 0
        pos = pos + 1;
        trig = -1;
    elseif a-b == -1 && trig == 0
        pos = pos -1;
        trig = 1;
    end

    if a == 1 && b == 1
        trig = 1;
    end
    p = pos;
end

== matlab function lab_1/Polling x6 ==
  data: a input; p output; b input
function p = fcn(a,b)
    persistent pos;
    persistent trigA;
    persistent trigB;
    if isempty(trigA)
        trigA = 1;
        trigB = 1;
        pos = 0;
    end
    if a-b == -1 && trigA
        pos = pos + 1;
        trigA = 2;
    elseif a-b == 1 && trigA
        pos = pos -1;
        trigA = 2;
    end


    if a-b == -1 && trigA == 0
        pos = pos + 1;
        trigA = -1;
    elseif a-b == 1 && trigA == 0
        pos = pos -1;
        trigA = -1;
    end


    if b-a == 1 && trigB
        pos = pos + 1;
        trigB = 2;
    elseif b-a == -1 && trigB
        pos = pos - 1;
        trigB = 2;
    end

    if b-a == 1 && trigB == 0
        pos = pos + 1;
        trigB = -1;
    elseif b-a == -1 && trigB == 0
        pos = pos - 1;
        trigB = -1;
    end

    if a == 0 && b == 0
        trigA = 0;
        trigB = 0;
    end

    if a == 1 && b == 1
        trigA = 1;
        trigB = 1;
    end
    p = pos;
end

== matlab function lab_1/QEI x3/MATLAB Function ==
  data: C output; P output; set input; cr input
function [C,P] = fcn(set,cr)
    persistent pr;
    persistent hom;
    persistent ps;
    max = 2048;

    if isempty(pr)
        pr = cr;
        hom = 0;
        ps = 0;
    end

    delta = cr - pr;

    if delta <= -1*(max/2)
        delta = delta + max + 1;
    elseif delta >= max/2
        delta = delta -max - 1;
    end

    if set
        hom = ps;
    end
    ps = ps + delta;
    C = ps - hom;
    pr = cr;
    P = C;
end

== matlab function lab_1/QEI x5/MATLAB Function ==
  data: C output; P output; set input; cr input
function [C,P] = fcn(set,cr)
    persistent pr;
    persistent hom;
    persistent ps;
    max = 2048;

    if isempty(pr)
        pr = cr;
        hom = 0;
        ps = 0;
    end

    delta = cr - pr;

    if delta <= -1*(max/2)
        delta = delta + max + 1;
    elseif delta >= max/2
        delta = delta -max - 1;
    end

    if set
        hom = ps;
    end
    ps = ps + delta;
    C = ps - hom;
    pr = cr;
    P = C;
end

== matlab function lab_1/QEI x6/MATLAB Function ==
  data: C output; P output; set input; cr input
function [C,P] = fcn(set,cr)
    persistent pr;
    persistent hom;
    persistent ps;
    max = 2048;

    if isempty(pr)
        pr = cr;
        hom = 0;
        ps = 0;
    end

    delta = cr - pr;

    if delta <= -1*(max/2)
        delta = delta + max + 1;
    elseif delta >= max/2
        delta = delta -max - 1;
    end

    if set
        hom = ps;
    end
    ps = ps + delta;
    C = ps - hom;
    pr = cr;
    P = C;
end

== stateflow chart lab_1/Chart1 ==
  state setup
    loop = 0;
    tic = 0;
    x_plot = 0;
    y_plot = 0;
  state set
    loop = 0;
  state loop1
    entry:
    tic = 1;
    during:
    loop = loop + 0.001;
    exit:
    tic = 0;
    x_plot = x_plot + 1
    y_plot = data
  (default) -> setup
  setup -> set
  loop1 -> set : [loop > 0.5 - 0.001]
  set -> loop1 : [input == 1]
  data: data input; input input; tic output; loop local; x_plot output; y_plot output

== stateflow chart lab_1/Chart2 ==
  state setup
    loop = 0;
    tic = 0;
    x_plot = 0;
    y_plot = 0;
  state set
    loop = 0;
  state loop1
    entry:
    tic = 1;
    during:
    loop = loop + 0.001;
    exit:
    tic = 0;
    x_plot = x_plot + 2.77778
    y_plot = data
  (default) -> setup
  setup -> set
  loop1 -> set : [loop > 0.5 - 0.001]
  set -> loop1 : [input == 1]
  data: data input; input input; tic output; loop local; x_plot output; y_plot output

== stateflow chart lab_1/Chart ==
  state setup
    loop = 0;
    tic = 0;
    x_plot = 0;
    y_plot = 0;
  state set
    loop = 0;
  state loop1
    entry:
    tic = 1;
    during:
    loop = loop + 0.001;
    exit:
    tic = 0;
    x_plot = x_plot + 10
    y_plot = data
  (default) -> setup
  setup -> set
  loop1 -> set : [loop > 0.5 - 0.001]
  set -> loop1 : [input == 1]
  data: data input; input input; tic output; loop local; x_plot output; y_plot output

== matlab function lab_1/Polling x1 ==
  data: a input; p output; b input
function p = fcn(a,b)
    persistent pos;
    persistent trig;
    if isempty(trig)
        trig = 1;
        pos = 0;
    end
    if a-b == -1 && trig
        pos = pos + 1;
        trig = 0;
    elseif a-b == 1 && trig
        pos = pos -1;
        trig = 0;
    end

    if a == 1 && b == 1
        trig = 1;
    end
    p = pos;
end

== matlab function lab_1/Polling x2 ==
  data: a input; p output; b input
function p = fcn(a,b)
    persistent pos;
    persistent trig;
    if isempty(trig)
        trig = 1;
        pos = 0;
    end
    if a-b == -1 && trig
        pos = pos + 1;
        trig = 2;
    elseif a-b == 1 && trig
        pos = pos -1;
        trig = 2;
    end

    if a == 0 && b == 0 
        trig = 0;
    end

    if a-b == 1 && trig == 0
        pos = pos + 1;
        trig = -1;
    elseif a-b == -1 && trig == 0
        pos = pos -1;
        trig = 1;
    end

    if a == 1 && b == 1
        trig = 1;
    end
    p = pos;
end

== matlab function lab_1/Polling x4 ==
  data: a input; p output; b input
function p = fcn(a,b)
    persistent pos;
    persistent trigA;
    persistent trigB;
    if isempty(trigA)
        trigA = 1;
        trigB = 1;
        pos = 0;
    end
    if a-b == -1 && trigA
        pos = pos + 1;
        trigA = 2;
    elseif a-b == 1 && trigA
        pos = pos -1;
        trigA = 2;
    end


    if a-b == -1 && trigA == 0
        pos = pos + 1;
        trigA = -1;
    elseif a-b == 1 && trigA == 0
        pos = pos -1;
        trigA = -1;
    end


    if b-a == 1 && trigB
        pos = pos + 1;
        trigB = 2;
    elseif b-a == -1 && trigB
        pos = pos - 1;
        trigB = 2;
    end

    if b-a == 1 && trigB == 0
        pos = pos + 1;
        trigB = -1;
    elseif b-a == -1 && trigB == 0
        pos = pos - 1;
        trigB = -1;
    end

    if a == 0 && b == 0
        trigA = 0;
        trigB = 0;
    end

    if a == 1 && b == 1
        trigA = 1;
        trigB = 1;
    end
    p = pos;
end

== matlab function lab_1/QEI x1/MATLAB Function ==
  data: max_cnt input; Count output; Pulse output; set input; curr input
function [Count,Pulse] = fcn(max_cnt,set,curr)
    persistent prev;
    persistent homing;
    persistent pos;

    if isempty(prev)
        prev = curr;
        homing = 0;
        pos = 0;
    end

    delta = curr - prev;

    if delta <= -1*(max_cnt/2)
        delta = delta + max_cnt + 1;
    elseif delta >= max_cnt/2
        delta = delta -max_cnt - 1;
    end

    if set
        homing = pos;
    end

    pos = pos + delta;
    Count = pos - homing;
    prev = curr;

    Pulse = Count;

end
